simulink model "EE238BuckBoostCon"  (R2018a)
settings: Solver=VariableStepAuto  StartTime=0.0  StopTime=0.065  MaxStep=1e-4  RelTol=1e-4  EnableMultiTasking=on
libraries: powerlib x13, powerlib_meascontrol x1
Description:
  | Copyright 2008-2018 The MathWorks, Inc.
settings Model: Creator=MathWorks  LastModifiedBy=Kishore Chatterjee
settings SolverCC: SolverResetMethod=Robust
settings OptimizationCC: EfficientFloat2IntCast=on  LifeSpan=inf
settings DebuggingCC: UniqueDataStoreMsg=error  StrictBusMsg=ErrorOnBusTreatedAsVector  SFUnexpectedBacktrackingDiag=warning  SFNoUnconditionalDefaultTransitionDiag=warning  SFExecutionAtInitializationDiag=none
settings CodeAppCC: StateflowObjectComments=on
settings GRTTargetCC: TargetLangStandard=C89/C90 (ANSI)  GeneratePreprocessorConditionals=Disable all
settings ConfigComp: CovMetricSettings=dw  CovHtmlReporting=on  CovSaveCumulativeToWorkspaceVar=on  CovSaveSingleToWorkspaceVar=on  CovExternalEMLEnable=off
settings SimscapeCC: SimscapeNormalizeSystem=off  SimscapeNominalValues={1, 'bar'; 1, 'cm^3/s'; 1, 'bar*kg/s'; 1, 'kJ/kg'; 1, 'kW'; }

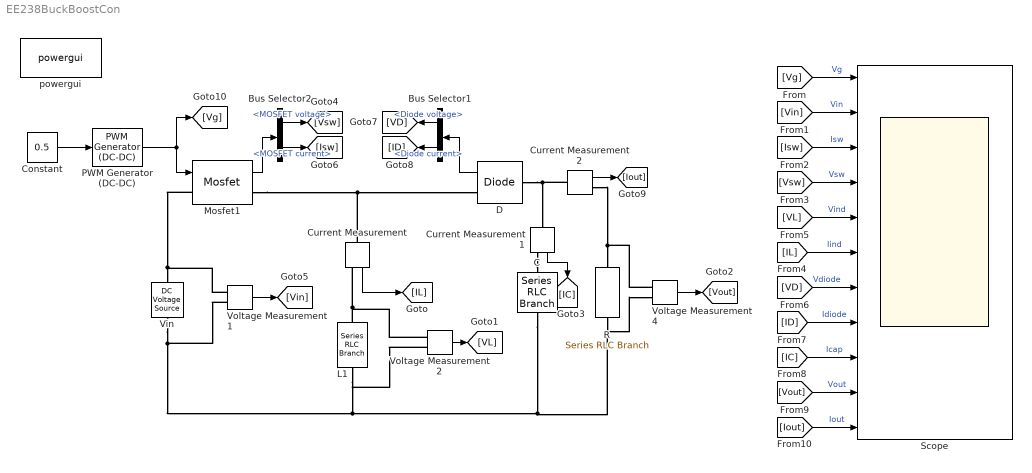
== system EE238BuckBoostCon ==
  Bus Selector1 : BusSelector  OutputSignals=Diode voltage,Diode current
  Bus Selector2 : BusSelector  OutputSignals=MOSFET voltage,MOSFET current
  C : powerlib/Elements/Series RLC Branch  LConnTagsString=__new0  RConnTagsString=__new0  BranchType=C  Resistance=1e-4  Inductance=200e-6  SetiL0=off  InitialCurrent=0  Capacitance=2000e-6  Setx0=on  InitialVoltage=0  Measurements=None
  Constant : Constant  Value=0.5
  Current Measurement : powerlib/Measurements/Current Measurement  PhasorSimulation=off  OutputType=Complex  PSBequivalent=0
  Current Measurement1 : powerlib/Measurements/Current Measurement  PhasorSimulation=off  OutputType=Complex  PSBequivalent=0
  Current Measurement2 : powerlib/Measurements/Current Measurement  PhasorSimulation=off  OutputType=Complex  PSBequivalent=0
  "D " : powerlib/Power Electronics/Diode  Ron=1e-3  Lon=0  Vf=0  IC=0  UseSnubber=off  Rs=inf  Cs=inf  Measurements=on
  L1 : powerlib/Elements/Series RLC Branch  LConnTagsString=__new0  RConnTagsString=__new0  BranchType=L  Resistance=1e-4  Inductance=750e-6  SetiL0=on  InitialCurrent=0  Capacitance=30e-6  Setx0=off  InitialVoltage=150  Measurements=None
  Mosfet1 : powerlib/Power Electronics/Mosfet  Ron=1e-3  Lon=0  Rd=1e-3  Vfd=0  IC=0  Rs=1e6  Cs=inf  Measurements=on
  PWM Generator (DC-DC) : powerlib_meascontrol/Pulse & Signal Generators/PWM Generator (DC-DC)  Fsw=5000  Ts=0
  R : powerlib/Elements/Series RLC Branch  LConnTagsString=__new0  RConnTagsString=__new0  BranchType=R  Resistance=1  Inductance=200e-6  SetiL0=off  InitialCurrent=0  Capacitance=400e-6  Setx0=off  InitialVoltage=0  Measurements=None
  Scope : Scope  NumInputPorts=11
  "Vin " : powerlib/Electrical Sources/DC Voltage Source  Amplitude=9  Measurements=None
  Voltage Measurement1 : powerlib/Measurements/Voltage Measurement  PhasorSimulation=off  OutputType=Complex  PSBequivalent=0
  Voltage Measurement2 : powerlib/Measurements/Voltage Measurement  PhasorSimulation=off  OutputType=Complex  PSBequivalent=0
  Voltage Measurement4 : powerlib/Measurements/Voltage Measurement  PhasorSimulation=off  OutputType=Complex  PSBequivalent=0
  powergui : powerlib/powergui  Priority=1  SimulationMode=Continuous  SampleTime=50e-6  frequency=60  Iterations=50  frequencyindice=0  Pbase=100e6  ErrMax=1e-4  UnitsV=kV  UnitsW=MW  buscounter=0  FunctionMessages=off  echomessages=off  EnableUseOfTLC=off  CurrentSourceSwitches=off  DisableSnubberDevices=off  DisableRonSwitches=off  DisableVfSwitches=off  DisplayEquations=off  SolverType=Tustin/Backward Euler (TBE)  Interpol=off  ExternalGateDelay=off  methode=off  Ts=100  x0status=blocks  SPID=on  SwTol=0  HookPort=off  RestoreLinks=warning  ResistiveCurrentMeasurement=off  Frange=[0:2:500]  Ylog=off  Xlog=on  ShowGrid=off  save=off  variable=ZData  structure=0  ZoomFFT=off  StartTime=0.0  cycles=1  DisplayStyle=1  fundamental=60  FreqAxis=off  MaxFrequency=1000  frequencyindicesteady=1  RmsSteady=1  display=off
  wires:
  Current Measurement/1 -> [IL]
  Voltage Measurement4/1 -> [Vout]
  Voltage Measurement1/1 -> [Vin]
  PWM Generator (DC-DC)/1 -> [Vg], Mosfet1/1
  Constant/1 -> PWM Generator (DC-DC)/1
  Voltage Measurement2/1 -> [VL]
  Current Measurement1/1 -> [IC]
  Current Measurement2/1 -> [Iout]
  [Vg] -> Scope/1  "Vg"
  [Vin] -> Scope/2  "Vin"
  [IL] -> Scope/6  "Iind"
  [VD] -> Scope/7  "Vdiode"
  [ID] -> Scope/8  "Idiode"
  [IC] -> Scope/9  "Icap"
  [Vout] -> Scope/10  "Vout"
  [Iout] -> Scope/11  "Iout"
  [VL] -> Scope/5  "Vind"
  Mosfet1/1 -> Bus Selector2/1
  Bus Selector2/1 -> [Vsw]  "<MOSFET voltage>"
  Bus Selector2/2 -> [Isw]  "<MOSFET current>"
  [Vsw] -> Scope/4  "Vsw"
  [Isw] -> Scope/3  "Isw"
  "D "/1 -> Bus Selector1/1
  Bus Selector1/1 -> [VD]  "<Diode voltage>"
  Bus Selector1/2 -> [ID]  "<Diode current>"
  connections:
  "Vin "/LConn1 -- Voltage Measurement2/LConn2 -- L1/RConn1 -- R/RConn1 -- Voltage Measurement4/LConn2 -- C/LConn1 -- Voltage Measurement1/LConn2
  "D "/LConn1 -- Current Measurement2/LConn1 -- Current Measurement1/LConn1
  Mosfet1/LConn1 -- Voltage Measurement1/LConn1 -- "Vin "/RConn1
  Current Measurement/LConn1 -- Mosfet1/RConn1 -- "D "/RConn1
  L1/LConn1 -- Voltage Measurement2/LConn1 -- Current Measurement/RConn1
  Current Measurement1/RConn1 -- C/RConn1
  Voltage Measurement4/LConn1 -- R/LConn1 -- Current Measurement2/RConn1
